simulink model "PulsePairProc_x4"  (Simulink 6.4)
settings: Solver=ode45  StartTime=0.0  StopTime=40000/12e6  RelTol=1e-3
libraries: xbsIndex_r4 x1049, simulink x4, dspsrcs4 x1
(part 1 of 8)
settings Model: LastModifiedBy=tbrimeye

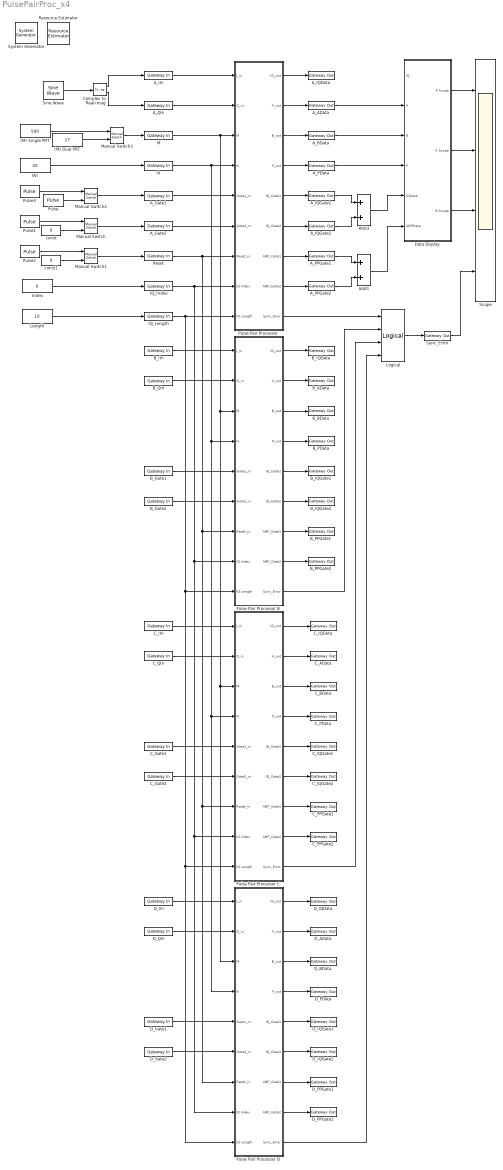
== system PulsePairProc_x4 ==
  " System Generator" : xbsIndex_r4/ System Generator  Tag=genX  SystemSampleTime=-1  xilinxfamily=Virtex4  part=xc4vlx60  speed=-11  package=ff668  synthesis_tool=XST  directory=C:/Work_Projects/Xilinx/SysGen_Outputs/PulsePairProcessor/PulsePairProc_x4_netlist  testbench=off  simulink_period=1/12e6  sysclk_period=(1/12e6)*1e9  incr_netlist=off  trim_vbits=Everywhere in SubSystem  dbl_ovrd=According to Block Masks  core_generation=According to Block Masks  run_coregen=off  deprecated_control=off  eval_field=0  block_type=sysgen
      settings: block_version=8.2
  (M) Dual PRT : Constant  Value=27  OutDataType=sfix(16)  ConRadixGroup=Use specified scaling  OutScaling=2^0  SampleTime=inf  FramePeriod=inf
  (M) Single PRT : Constant  Value=500  OutDataType=sfix(16)  ConRadixGroup=Use specified scaling  OutScaling=2^0  SampleTime=inf  FramePeriod=inf
  (N) : Constant  Value=20  OutDataType=sfix(16)  ConRadixGroup=Use specified scaling  OutScaling=2^0  SampleTime=inf  FramePeriod=inf
  A_AData : xbsIndex_r4/Gateway Out  hdl_port=on  timing_constraint=None  locs_specified=off  LOCs={}  block_type=gatewayout
      settings: infoedit="Gateway out block.  Converts Xilinx fixed point inputs into ouputs of type Simulink integer, double, or fixed point.<P><P>Hardware notes:  In hardware these blocks become top level output ports or are discarded, depending on how they are configured."  xl_area=[0 0 0 0 32 0 0]  block_version=8.2
  A_BData : xbsIndex_r4/Gateway Out  hdl_port=on  timing_constraint=None  locs_specified=off  LOCs={}  block_type=gatewayout
      settings: infoedit="Gateway out block.  Converts Xilinx fixed point inputs into ouputs of type Simulink integer, double, or fixed point.<P><P>Hardware notes:  In hardware these blocks become top level output ports or are discarded, depending on how they are configured."  xl_area=[0 0 0 0 32 0 0]  block_version=8.2
  A_Gate1 : xbsIndex_r4/Gateway In  arith_type=Boolean  n_bits=18  bin_pt=0  quantization="Round  (unbiased: +/- Inf)"  overflow=Flag as error  period=1/12e6  dbl_ovrd=off  timing_constraint=None  locs_specified=off  LOCs={}  block_type=gatewayin
      settings: infoedit="Gateway in block.  Converts inputs of type Simulink integer, double and fixed point to  Xilinx fixed point type.<P><P>Hardware notes:  In hardware these blocks become top level input ports."  xl_area=[0 0 0 0 1 0 0]  block_version=8.2
  A_Gate2 : xbsIndex_r4/Gateway In  arith_type=Boolean  n_bits=18  bin_pt=0  quantization="Round  (unbiased: +/- Inf)"  overflow=Flag as error  period=1/12e6  dbl_ovrd=off  timing_constraint=None  locs_specified=off  LOCs={}  block_type=gatewayin
      settings: infoedit="Gateway in block.  Converts inputs of type Simulink integer, double and fixed point to  Xilinx fixed point type.<P><P>Hardware notes:  In hardware these blocks become top level input ports."  xl_area=[0 0 0 0 1 0 0]  block_version=8.2
  A_IIn : xbsIndex_r4/Gateway In  arith_type="Signed  (2's comp)"  n_bits=16  bin_pt=15  quantization="Round  (unbiased: +/- Inf)"  overflow=Saturate  period=1/12e6  dbl_ovrd=off  timing_constraint=None  locs_specified=off  LOCs={}  block_type=gatewayin
      settings: infoedit="Gateway in block.  Converts inputs of type Simulink integer, double and fixed point to  Xilinx fixed point type.<P><P>Hardware notes:  In hardware these blocks become top level input ports."  xl_area=[0 0 0 0 16 0 0]  block_version=8.2
  A_IQData : xbsIndex_r4/Gateway Out  hdl_port=on  timing_constraint=None  locs_specified=off  LOCs={}  block_type=gatewayout
      settings: infoedit="Gateway out block.  Converts Xilinx fixed point inputs into ouputs of type Simulink integer, double, or fixed point.<P><P>Hardware notes:  In hardware these blocks become top level output ports or are discarded, depending on how they are configured."  xl_area=[0 0 0 0 32 0 0]  block_version=8.2
  A_IQGate1 : xbsIndex_r4/Gateway Out  hdl_port=on  timing_constraint=None  locs_specified=off  LOCs={}  block_type=gatewayout
      settings: infoedit="Gateway out block.  Converts Xilinx fixed point inputs into ouputs of type Simulink integer, double, or fixed point.<P><P>Hardware notes:  In hardware these blocks become top level output ports or are discarded, depending on how they are configured."  xl_area=[0 0 0 0 32 0 0]  block_version=8.2
  A_IQGate2 : xbsIndex_r4/Gateway Out  hdl_port=on  timing_constraint=None  locs_specified=off  LOCs={}  block_type=gatewayout
      settings: infoedit="Gateway out block.  Converts Xilinx fixed point inputs into ouputs of type Simulink integer, double, or fixed point.<P><P>Hardware notes:  In hardware these blocks become top level output ports or are discarded, depending on how they are configured."  xl_area=[0 0 0 0 32 0 0]  block_version=8.2
  A_PData : xbsIndex_r4/Gateway Out  hdl_port=on  timing_constraint=None  locs_specified=off  LOCs={}  block_type=gatewayout
      settings: infoedit="Gateway out block.  Converts Xilinx fixed point inputs into ouputs of type Simulink integer, double, or fixed point.<P><P>Hardware notes:  In hardware these blocks become top level output ports or are discarded, depending on how they are configured."  xl_area=[0 0 0 0 32 0 0]  block_version=8.2
  A_PPGate1 : xbsIndex_r4/Gateway Out  hdl_port=on  timing_constraint=None  locs_specified=off  LOCs={}  block_type=gatewayout
      settings: infoedit="Gateway out block.  Converts Xilinx fixed point inputs into ouputs of type Simulink integer, double, or fixed point.<P><P>Hardware notes:  In hardware these blocks become top level output ports or are discarded, depending on how they are configured."  xl_area=[0 0 0 0 32 0 0]  block_version=8.2
  A_PPGate2 : xbsIndex_r4/Gateway Out  hdl_port=on  timing_constraint=None  locs_specified=off  LOCs={}  block_type=gatewayout
      settings: infoedit="Gateway out block.  Converts Xilinx fixed point inputs into ouputs of type Simulink integer, double, or fixed point.<P><P>Hardware notes:  In hardware these blocks become top level output ports or are discarded, depending on how they are configured."  xl_area=[0 0 0 0 32 0 0]  block_version=8.2
  A_QIn : xbsIndex_r4/Gateway In  arith_type="Signed  (2's comp)"  n_bits=16  bin_pt=15  quantization="Round  (unbiased: +/- Inf)"  overflow=Saturate  period=1/12e6  dbl_ovrd=off  timing_constraint=None  locs_specified=off  LOCs={}  block_type=gatewayin
      settings: infoedit="Gateway in block.  Converts inputs of type Simulink integer, double and fixed point to  Xilinx fixed point type.<P><P>Hardware notes:  In hardware these blocks become top level input ports."  xl_area=[0 0 0 0 16 0 0]  block_version=8.2
  Add1 : Sum  OutScaling=2^-10
  Add3 : Sum  OutScaling=2^-10
  B_AData : xbsIndex_r4/Gateway Out  hdl_port=on  timing_constraint=None  locs_specified=off  LOCs={}  block_type=gatewayout
      settings: infoedit="Gateway out block.  Converts Xilinx fixed point inputs into ouputs of type Simulink integer, double, or fixed point.<P><P>Hardware notes:  In hardware these blocks become top level output ports or are discarded, depending on how they are configured."  xl_area=[0 0 0 0 32 0 0]  block_version=8.2
  B_BData : xbsIndex_r4/Gateway Out  hdl_port=on  timing_constraint=None  locs_specified=off  LOCs={}  block_type=gatewayout
      settings: infoedit="Gateway out block.  Converts Xilinx fixed point inputs into ouputs of type Simulink integer, double, or fixed point.<P><P>Hardware notes:  In hardware these blocks become top level output ports or are discarded, depending on how they are configured."  xl_area=[0 0 0 0 32 0 0]  block_version=8.2
  B_Gate1 : xbsIndex_r4/Gateway In  arith_type=Boolean  n_bits=18  bin_pt=0  quantization="Round  (unbiased: +/- Inf)"  overflow=Flag as error  period=1/12e6  dbl_ovrd=off  timing_constraint=None  locs_specified=off  LOCs={}  block_type=gatewayin
      settings: infoedit="Gateway in block.  Converts inputs of type Simulink integer, double and fixed point to  Xilinx fixed point type.<P><P>Hardware notes:  In hardware these blocks become top level input ports."  xl_area=[0 0 0 0 1 0 0]  block_version=8.2
  B_Gate2 : xbsIndex_r4/Gateway In  arith_type=Boolean  n_bits=18  bin_pt=0  quantization="Round  (unbiased: +/- Inf)"  overflow=Flag as error  period=1/12e6  dbl_ovrd=off  timing_constraint=None  locs_specified=off  LOCs={}  block_type=gatewayin
      settings: infoedit="Gateway in block.  Converts inputs of type Simulink integer, double and fixed point to  Xilinx fixed point type.<P><P>Hardware notes:  In hardware these blocks become top level input ports."  xl_area=[0 0 0 0 1 0 0]  block_version=8.2
  B_IIn : xbsIndex_r4/Gateway In  arith_type="Signed  (2's comp)"  n_bits=16  bin_pt=15  quantization="Round  (unbiased: +/- Inf)"  overflow=Saturate  period=1/12e6  dbl_ovrd=off  timing_constraint=None  locs_specified=off  LOCs={}  block_type=gatewayin
      settings: infoedit="Gateway in block.  Converts inputs of type Simulink integer, double and fixed point to  Xilinx fixed point type.<P><P>Hardware notes:  In hardware these blocks become top level input ports."  xl_area=[0 0 0 0 16 0 0]  block_version=8.2
  B_IQData : xbsIndex_r4/Gateway Out  hdl_port=on  timing_constraint=None  locs_specified=off  LOCs={}  block_type=gatewayout
      settings: infoedit="Gateway out block.  Converts Xilinx fixed point inputs into ouputs of type Simulink integer, double, or fixed point.<P><P>Hardware notes:  In hardware these blocks become top level output ports or are discarded, depending on how they are configured."  xl_area=[0 0 0 0 32 0 0]  block_version=8.2
  B_IQGate1 : xbsIndex_r4/Gateway Out  hdl_port=on  timing_constraint=None  locs_specified=off  LOCs={}  block_type=gatewayout
      settings: infoedit="Gateway out block.  Converts Xilinx fixed point inputs into ouputs of type Simulink integer, double, or fixed point.<P><P>Hardware notes:  In hardware these blocks become top level output ports or are discarded, depending on how they are configured."  xl_area=[0 0 0 0 32 0 0]  block_version=8.2
  B_IQGate2 : xbsIndex_r4/Gateway Out  hdl_port=on  timing_constraint=None  locs_specified=off  LOCs={}  block_type=gatewayout
      settings: infoedit="Gateway out block.  Converts Xilinx fixed point inputs into ouputs of type Simulink integer, double, or fixed point.<P><P>Hardware notes:  In hardware these blocks become top level output ports or are discarded, depending on how they are configured."  xl_area=[0 0 0 0 32 0 0]  block_version=8.2
  B_PData : xbsIndex_r4/Gateway Out  hdl_port=on  timing_constraint=None  locs_specified=off  LOCs={}  block_type=gatewayout
      settings: infoedit="Gateway out block.  Converts Xilinx fixed point inputs into ouputs of type Simulink integer, double, or fixed point.<P><P>Hardware notes:  In hardware these blocks become top level output ports or are discarded, depending on how they are configured."  xl_area=[0 0 0 0 32 0 0]  block_version=8.2
  B_PPGate1 : xbsIndex_r4/Gateway Out  hdl_port=on  timing_constraint=None  locs_specified=off  LOCs={}  block_type=gatewayout
      settings: infoedit="Gateway out block.  Converts Xilinx fixed point inputs into ouputs of type Simulink integer, double, or fixed point.<P><P>Hardware notes:  In hardware these blocks become top level output ports or are discarded, depending on how they are configured."  xl_area=[0 0 0 0 32 0 0]  block_version=8.2
  B_PPGate2 : xbsIndex_r4/Gateway Out  hdl_port=on  timing_constraint=None  locs_specified=off  LOCs={}  block_type=gatewayout
      settings: infoedit="Gateway out block.  Converts Xilinx fixed point inputs into ouputs of type Simulink integer, double, or fixed point.<P><P>Hardware notes:  In hardware these blocks become top level output ports or are discarded, depending on how they are configured."  xl_area=[0 0 0 0 32 0 0]  block_version=8.2
  B_QIn : xbsIndex_r4/Gateway In  arith_type="Signed  (2's comp)"  n_bits=16  bin_pt=15  quantization="Round  (unbiased: +/- Inf)"  overflow=Saturate  period=1/12e6  dbl_ovrd=off  timing_constraint=None  locs_specified=off  LOCs={}  block_type=gatewayin
      settings: infoedit="Gateway in block.  Converts inputs of type Simulink integer, double and fixed point to  Xilinx fixed point type.<P><P>Hardware notes:  In hardware these blocks become top level input ports."  xl_area=[0 0 0 0 16 0 0]  block_version=8.2
  C_AData : xbsIndex_r4/Gateway Out  hdl_port=on  timing_constraint=None  locs_specified=off  LOCs={}  block_type=gatewayout
      settings: infoedit="Gateway out block.  Converts Xilinx fixed point inputs into ouputs of type Simulink integer, double, or fixed point.<P><P>Hardware notes:  In hardware these blocks become top level output ports or are discarded, depending on how they are configured."  xl_area=[0 0 0 0 32 0 0]  block_version=8.2
  C_BData : xbsIndex_r4/Gateway Out  hdl_port=on  timing_constraint=None  locs_specified=off  LOCs={}  block_type=gatewayout
      settings: infoedit="Gateway out block.  Converts Xilinx fixed point inputs into ouputs of type Simulink integer, double, or fixed point.<P><P>Hardware notes:  In hardware these blocks become top level output ports or are discarded, depending on how they are configured."  xl_area=[0 0 0 0 32 0 0]  block_version=8.2
  C_Gate1 : xbsIndex_r4/Gateway In  arith_type=Boolean  n_bits=18  bin_pt=0  quantization="Round  (unbiased: +/- Inf)"  overflow=Flag as error  period=1/12e6  dbl_ovrd=off  timing_constraint=None  locs_specified=off  LOCs={}  block_type=gatewayin
      settings: infoedit="Gateway in block.  Converts inputs of type Simulink integer, double and fixed point to  Xilinx fixed point type.<P><P>Hardware notes:  In hardware these blocks become top level input ports."  xl_area=[0 0 0 0 1 0 0]  block_version=8.2
  C_Gate2 : xbsIndex_r4/Gateway In  arith_type=Boolean  n_bits=18  bin_pt=0  quantization="Round  (unbiased: +/- Inf)"  overflow=Flag as error  period=1/12e6  dbl_ovrd=off  timing_constraint=None  locs_specified=off  LOCs={}  block_type=gatewayin
      settings: infoedit="Gateway in block.  Converts inputs of type Simulink integer, double and fixed point to  Xilinx fixed point type.<P><P>Hardware notes:  In hardware these blocks become top level input ports."  xl_area=[0 0 0 0 1 0 0]  block_version=8.2
  C_IIn : xbsIndex_r4/Gateway In  arith_type="Signed  (2's comp)"  n_bits=16  bin_pt=15  quantization="Round  (unbiased: +/- Inf)"  overflow=Saturate  period=1/12e6  dbl_ovrd=off  timing_constraint=None  locs_specified=off  LOCs={}  block_type=gatewayin
      settings: infoedit="Gateway in block.  Converts inputs of type Simulink integer, double and fixed point to  Xilinx fixed point type.<P><P>Hardware notes:  In hardware these blocks become top level input ports."  xl_area=[0 0 0 0 16 0 0]  block_version=8.2
  C_IQData : xbsIndex_r4/Gateway Out  hdl_port=on  timing_constraint=None  locs_specified=off  LOCs={}  block_type=gatewayout
      settings: infoedit="Gateway out block.  Converts Xilinx fixed point inputs into ouputs of type Simulink integer, double, or fixed point.<P><P>Hardware notes:  In hardware these blocks become top level output ports or are discarded, depending on how they are configured."  xl_area=[0 0 0 0 32 0 0]  block_version=8.2
  C_IQGate1 : xbsIndex_r4/Gateway Out  hdl_port=on  timing_constraint=None  locs_specified=off  LOCs={}  block_type=gatewayout
      settings: infoedit="Gateway out block.  Converts Xilinx fixed point inputs into ouputs of type Simulink integer, double, or fixed point.<P><P>Hardware notes:  In hardware these blocks become top level output ports or are discarded, depending on how they are configured."  xl_area=[0 0 0 0 32 0 0]  block_version=8.2
  C_IQGate2 : xbsIndex_r4/Gateway Out  hdl_port=on  timing_constraint=None  locs_specified=off  LOCs={}  block_type=gatewayout
      settings: infoedit="Gateway out block.  Converts Xilinx fixed point inputs into ouputs of type Simulink integer, double, or fixed point.<P><P>Hardware notes:  In hardware these blocks become top level output ports or are discarded, depending on how they are configured."  xl_area=[0 0 0 0 32 0 0]  block_version=8.2
  C_PData : xbsIndex_r4/Gateway Out  hdl_port=on  timing_constraint=None  locs_specified=off  LOCs={}  block_type=gatewayout
      settings: infoedit="Gateway out block.  Converts Xilinx fixed point inputs into ouputs of type Simulink integer, double, or fixed point.<P><P>Hardware notes:  In hardware these blocks become top level output ports or are discarded, depending on how they are configured."  xl_area=[0 0 0 0 32 0 0]  block_version=8.2
  C_PPGate1 : xbsIndex_r4/Gateway Out  hdl_port=on  timing_constraint=None  locs_specified=off  LOCs={}  block_type=gatewayout
      settings: infoedit="Gateway out block.  Converts Xilinx fixed point inputs into ouputs of type Simulink integer, double, or fixed point.<P><P>Hardware notes:  In hardware these blocks become top level output ports or are discarded, depending on how they are configured."  xl_area=[0 0 0 0 32 0 0]  block_version=8.2
  C_PPGate2 : xbsIndex_r4/Gateway Out  hdl_port=on  timing_constraint=None  locs_specified=off  LOCs={}  block_type=gatewayout
      settings: infoedit="Gateway out block.  Converts Xilinx fixed point inputs into ouputs of type Simulink integer, double, or fixed point.<P><P>Hardware notes:  In hardware these blocks become top level output ports or are discarded, depending on how they are configured."  xl_area=[0 0 0 0 32 0 0]  block_version=8.2
  C_QIn : xbsIndex_r4/Gateway In  arith_type="Signed  (2's comp)"  n_bits=16  bin_pt=15  quantization="Round  (unbiased: +/- Inf)"  overflow=Saturate  period=1/12e6  dbl_ovrd=off  timing_constraint=None  locs_specified=off  LOCs={}  block_type=gatewayin
      settings: infoedit="Gateway in block.  Converts inputs of type Simulink integer, double and fixed point to  Xilinx fixed point type.<P><P>Hardware notes:  In hardware these blocks become top level input ports."  xl_area=[0 0 0 0 16 0 0]  block_version=8.2
  Complex to Real-Imag : ComplexToRealImag
  D_AData : xbsIndex_r4/Gateway Out  hdl_port=on  timing_constraint=None  locs_specified=off  LOCs={}  block_type=gatewayout
      settings: infoedit="Gateway out block.  Converts Xilinx fixed point inputs into ouputs of type Simulink integer, double, or fixed point.<P><P>Hardware notes:  In hardware these blocks become top level output ports or are discarded, depending on how they are configured."  xl_area=[0 0 0 0 32 0 0]  block_version=8.2
  D_BData : xbsIndex_r4/Gateway Out  hdl_port=on  timing_constraint=None  locs_specified=off  LOCs={}  block_type=gatewayout
      settings: infoedit="Gateway out block.  Converts Xilinx fixed point inputs into ouputs of type Simulink integer, double, or fixed point.<P><P>Hardware notes:  In hardware these blocks become top level output ports or are discarded, depending on how they are configured."  xl_area=[0 0 0 0 32 0 0]  block_version=8.2
  D_Gate1 : xbsIndex_r4/Gateway In  arith_type=Boolean  n_bits=18  bin_pt=0  quantization="Round  (unbiased: +/- Inf)"  overflow=Flag as error  period=1/12e6  dbl_ovrd=off  timing_constraint=None  locs_specified=off  LOCs={}  block_type=gatewayin
      settings: infoedit="Gateway in block.  Converts inputs of type Simulink integer, double and fixed point to  Xilinx fixed point type.<P><P>Hardware notes:  In hardware these blocks become top level input ports."  xl_area=[0 0 0 0 1 0 0]  block_version=8.2
  D_Gate2 : xbsIndex_r4/Gateway In  arith_type=Boolean  n_bits=18  bin_pt=0  quantization="Round  (unbiased: +/- Inf)"  overflow=Flag as error  period=1/12e6  dbl_ovrd=off  timing_constraint=None  locs_specified=off  LOCs={}  block_type=gatewayin
      settings: infoedit="Gateway in block.  Converts inputs of type Simulink integer, double and fixed point to  Xilinx fixed point type.<P><P>Hardware notes:  In hardware these blocks become top level input ports."  xl_area=[0 0 0 0 1 0 0]  block_version=8.2
  D_IIn : xbsIndex_r4/Gateway In  arith_type="Signed  (2's comp)"  n_bits=16  bin_pt=15  quantization="Round  (unbiased: +/- Inf)"  overflow=Saturate  period=1/12e6  dbl_ovrd=off  timing_constraint=None  locs_specified=off  LOCs={}  block_type=gatewayin
      settings: infoedit="Gateway in block.  Converts inputs of type Simulink integer, double and fixed point to  Xilinx fixed point type.<P><P>Hardware notes:  In hardware these blocks become top level input ports."  xl_area=[0 0 0 0 16 0 0]  block_version=8.2
  D_IQData : xbsIndex_r4/Gateway Out  hdl_port=on  timing_constraint=None  locs_specified=off  LOCs={}  block_type=gatewayout
      settings: infoedit="Gateway out block.  Converts Xilinx fixed point inputs into ouputs of type Simulink integer, double, or fixed point.<P><P>Hardware notes:  In hardware these blocks become top level output ports or are discarded, depending on how they are configured."  xl_area=[0 0 0 0 32 0 0]  block_version=8.2
  D_IQGate1 : xbsIndex_r4/Gateway Out  hdl_port=on  timing_constraint=None  locs_specified=off  LOCs={}  block_type=gatewayout
      settings: infoedit="Gateway out block.  Converts Xilinx fixed point inputs into ouputs of type Simulink integer, double, or fixed point.<P><P>Hardware notes:  In hardware these blocks become top level output ports or are discarded, depending on how they are configured."  xl_area=[0 0 0 0 32 0 0]  block_version=8.2
  D_IQGate2 : xbsIndex_r4/Gateway Out  hdl_port=on  timing_constraint=None  locs_specified=off  LOCs={}  block_type=gatewayout
      settings: infoedit="Gateway out block.  Converts Xilinx fixed point inputs into ouputs of type Simulink integer, double, or fixed point.<P><P>Hardware notes:  In hardware these blocks become top level output ports or are discarded, depending on how they are configured."  xl_area=[0 0 0 0 32 0 0]  block_version=8.2
  D_PData : xbsIndex_r4/Gateway Out  hdl_port=on  timing_constraint=None  locs_specified=off  LOCs={}  block_type=gatewayout
      settings: infoedit="Gateway out block.  Converts Xilinx fixed point inputs into ouputs of type Simulink integer, double, or fixed point.<P><P>Hardware notes:  In hardware these blocks become top level output ports or are discarded, depending on how they are configured."  xl_area=[0 0 0 0 32 0 0]  block_version=8.2
  D_PPGate1 : xbsIndex_r4/Gateway Out  hdl_port=on  timing_constraint=None  locs_specified=off  LOCs={}  block_type=gatewayout
      settings: infoedit="Gateway out block.  Converts Xilinx fixed point inputs into ouputs of type Simulink integer, double, or fixed point.<P><P>Hardware notes:  In hardware these blocks become top level output ports or are discarded, depending on how they are configured."  xl_area=[0 0 0 0 32 0 0]  block_version=8.2
  D_PPGate2 : xbsIndex_r4/Gateway Out  hdl_port=on  timing_constraint=None  locs_specified=off  LOCs={}  block_type=gatewayout
      settings: infoedit="Gateway out block.  Converts Xilinx fixed point inputs into ouputs of type Simulink integer, double, or fixed point.<P><P>Hardware notes:  In hardware these blocks become top level output ports or are discarded, depending on how they are configured."  xl_area=[0 0 0 0 32 0 0]  block_version=8.2
  D_QIn : xbsIndex_r4/Gateway In  arith_type="Signed  (2's comp)"  n_bits=16  bin_pt=15  quantization="Round  (unbiased: +/- Inf)"  overflow=Saturate  period=1/12e6  dbl_ovrd=off  timing_constraint=None  locs_specified=off  LOCs={}  block_type=gatewayin
      settings: infoedit="Gateway in block.  Converts inputs of type Simulink integer, double and fixed point to  Xilinx fixed point type.<P><P>Hardware notes:  In hardware these blocks become top level input ports."  xl_area=[0 0 0 0 16 0 0]  block_version=8.2
  Data Display : Subsystem
  IQ_Index : xbsIndex_r4/Gateway In  arith_type=Unsigned  n_bits=10  bin_pt=0  quantization="Round  (unbiased: +/- Inf)"  overflow=Flag as error  period=1/12e6  dbl_ovrd=off  timing_constraint=None  locs_specified=off  LOCs={}  block_type=gatewayin
      settings: infoedit="Gateway in block.  Converts inputs of type Simulink integer, double and fixed point to  Xilinx fixed point type.<P><P>Hardware notes:  In hardware these blocks become top level input ports."  xl_area=[0 0 0 0 11 0 0]  block_version=8.2
  IQ_Length : xbsIndex_r4/Gateway In  arith_type=Unsigned  n_bits=10  bin_pt=0  quantization="Round  (unbiased: +/- Inf)"  overflow=Flag as error  period=1/12e6  dbl_ovrd=off  timing_constraint=None  locs_specified=off  LOCs={}  block_type=gatewayin
      settings: infoedit="Gateway in block.  Converts inputs of type Simulink integer, double and fixed point to  Xilinx fixed point type.<P><P>Hardware notes:  In hardware these blocks become top level input ports."  xl_area=[0 0 0 0 11 0 0]  block_version=8.2
  Index : Constant  Value=0  OutDataType=sfix(16)  ConRadixGroup=Use specified scaling  OutScaling=2^0  SampleTime=inf  FramePeriod=inf
  Length : Constant  Value=10  OutDataType=sfix(16)  ConRadixGroup=Use specified scaling  OutScaling=2^0  SampleTime=inf  FramePeriod=inf
  Logical : xbsIndex_r4/Logical  logical_function=OR  inputs=4  en=off  latency=0  precision=Full  arith_type=Unsigned  n_bits=16  bin_pt=0  align_bp=on  dbl_ovrd=off  block_type=logical
      settings: block_version=8.2
  M : xbsIndex_r4/Gateway In  arith_type=Unsigned  n_bits=10  bin_pt=0  quantization="Round  (unbiased: +/- Inf)"  overflow=Flag as error  period=1/12e6  dbl_ovrd=off  timing_constraint=None  locs_specified=off  LOCs={}  block_type=gatewayin
      settings: infoedit="Gateway in block.  Converts inputs of type Simulink integer, double and fixed point to  Xilinx fixed point type.<P><P>Hardware notes:  In hardware these blocks become top level input ports."  xl_area=[0 0 0 0 11 0 0]  block_version=8.2
  Manual Switch : simulink/Signal Routing/Manual Switch  SystemSampleTime=-1  sw=0  action=0
  Manual Switch1 : simulink/Signal Routing/Manual Switch  SystemSampleTime=-1  sw=0  action=0
  Manual Switch2 : simulink/Signal Routing/Manual Switch  SystemSampleTime=-1  sw=1  action=0
  Manual Switch3 : simulink/Signal Routing/Manual Switch  SystemSampleTime=-1  sw=1  action=0
  N : xbsIndex_r4/Gateway In  arith_type=Unsigned  n_bits=7  bin_pt=0  quantization="Round  (unbiased: +/- Inf)"  overflow=Flag as error  period=1/12e6  dbl_ovrd=off  timing_constraint=None  locs_specified=off  LOCs={}  block_type=gatewayin
      settings: infoedit="Gateway in block.  Converts inputs of type Simulink integer, double and fixed point to  Xilinx fixed point type.<P><P>Hardware notes:  In hardware these blocks become top level input ports."  xl_area=[0 0 0 0 7 0 0]  block_version=8.2
  Pulse : DiscretePulseGenerator  PulseType=Time based  Period=900/40e6  PulseWidth=10  PhaseDelay=0*100/12e6
  Pulse Pair Processor : Subsystem
  Pulse Pair Processor B : Subsystem
  Pulse Pair Processor C : Subsystem
  Pulse Pair Processor D : Subsystem
  Pulse1 : DiscretePulseGenerator  PulseType=Time based  Period=900/40e6  PulseWidth=10  PhaseDelay=150/12e6
  Pulse2 : DiscretePulseGenerator  PulseType=Time based  Period=5000/12e6  PhaseDelay=600/12e6
  Pulse3 : DiscretePulseGenerator  PulseType=Time based  Period=625/12e6  PulseWidth=80  PhaseDelay=0/12e6
  Reset : xbsIndex_r4/Gateway In  arith_type=Boolean  n_bits=18  bin_pt=0  quantization="Round  (unbiased: +/- Inf)"  overflow=Flag as error  period=1/12e6  dbl_ovrd=off  timing_constraint=None  locs_specified=off  LOCs={}  block_type=gatewayin
      settings: infoedit="Gateway in block.  Converts inputs of type Simulink integer, double and fixed point to  Xilinx fixed point type.<P><P>Hardware notes:  In hardware these blocks become top level input ports."  xl_area=[0 0 0 0 1 0 0]  block_version=8.2
  Resource Estimator : xbsIndex_r4/Resource Estimator  Tag=resEstTag  Slices=813  FFs=745  BRAMs=24  LUTs=1307  IOBs=244  EBMs=6  TBUFs=0  xl_use_estimator_area=off  est_options=Post Map  xl_estimator_area=[1915 2342 0 3405 33 4 0]  block_type=resource_estimator
      settings: AttributesFormatString=Resource\nEstimator  block_version=8.2
  Scope : Scope  NumInputPorts=4
      settings: TimeRange=0.0002083333333333334  YMin=-1~-5~-5~-5  YMax=1~5~5~5  MaxDataPoints=5000000
  Sine Wave : dspsrcs4/Sine Wave  Amplitude=.99  Frequency=10e3  Phase=0  SampleMode=Discrete  OutComplex=Complex  CompMethod=Trigonometric fcn  TableSize=Speed  SampleTime=1/12e6  SamplesPerFrame=1  dataType=double  wordLen=16  udDataType=sfix(16)  fracBitsMode=Best precision  numFracBits=15  ResetState=Restart at time zero
  Sync_Error : xbsIndex_r4/Gateway Out  hdl_port=on  timing_constraint=None  locs_specified=off  LOCs={}  block_type=gatewayout
      settings: infoedit="Gateway out block.  Converts Xilinx fixed point inputs into ouputs of type Simulink integer, double, or fixed point.<P><P>Hardware notes:  In hardware these blocks become top level output ports or are discarded, depending on how they are configured."  xl_area=[0 0 0 0 32 0 0]  block_version=8.2
  const : Constant  Value=0  OutDataType=sfix(16)  ConRadixGroup=Use specified scaling  OutScaling=2^0  SampleTime=inf  FramePeriod=inf
  const1 : Constant  Value=0  OutDataType=sfix(16)  ConRadixGroup=Use specified scaling  OutScaling=2^0  SampleTime=inf  FramePeriod=inf
  wires:
  A_IIn/1 -> Pulse Pair Processor/1(I_in)
  A_QIn/1 -> Pulse Pair Processor/2(Q_in)
  (N)/1 -> N/1
  M/1 -> Pulse Pair Processor D/3(M), Pulse Pair Processor C/3(M), Pulse Pair Processor B/3(M), Pulse Pair Processor/3(M)
  N/1 -> Pulse Pair Processor D/4(N), Pulse Pair Processor C/4(N), Pulse Pair Processor B/4(N), Pulse Pair Processor/4(N)
  Pulse1/1 -> Manual Switch/1
  const/1 -> Manual Switch/2
  Manual Switch/1 -> A_Gate2/1
  A_Gate1/1 -> Pulse Pair Processor/5(Gate1_in)
  A_Gate2/1 -> Pulse Pair Processor/6(Gate2_in)
  Pulse Pair Processor/2(A_out) -> A_AData/1
  Pulse Pair Processor/3(B_out) -> A_BData/1
  Pulse Pair Processor/4(P_out) -> A_PData/1
  Data Display/1(P Scope) -> Scope/1
  Data Display/2(A Scope) -> Scope/2
  Data Display/3(B Scope) -> Scope/3
  Pulse Pair Processor/1(IQ_out) -> A_IQData/1
  Pulse Pair Processor/5(IQ_Gate1) -> A_IQGate1/1
  Pulse Pair Processor/6(IQ_Gate2) -> A_IQGate2/1
  A_IQGate1/1 -> Add3/1
  A_IQGate2/1 -> Add3/2
  Pulse Pair Processor/7(ABP_Gate1) -> A_PPGate1/1
  Pulse Pair Processor/8(ABP_Gate2) -> A_PPGate2/1
  A_PData/1 -> Data Display/4(P)
  Reset/1 -> Pulse Pair Processor D/7(Reset_in), Pulse Pair Processor C/7(Reset_in), Pulse Pair Processor B/7(Reset_in), Pulse Pair Processor/7(Reset_in)
  Pulse2/1 -> Manual Switch1/1
  const1/1 -> Manual Switch1/2
  Manual Switch1/1 -> Reset/1
  A_AData/1 -> Data Display/2(A)
  A_BData/1 -> Data Display/3(B)
  A_PPGate1/1 -> Add1/1
  A_PPGate2/1 -> Add1/2
  Add1/1 -> Data Display/6(ABPGate)
  Sine Wave/1 -> Complex to Real-Imag/1
  Complex to Real-Imag/1 -> A_IIn/1
  Complex to Real-Imag/2 -> A_QIn/1
  Add3/1 -> Data Display/5(IQGate)
  IQ_Index/1 -> Pulse Pair Processor D/8(IQ Index), Pulse Pair Processor C/8(IQ Index), Pulse Pair Processor B/8(IQ Index), Pulse Pair Processor/8(IQ Index)
  IQ_Length/1 -> Pulse Pair Processor D/9(IQ Length), Pulse Pair Processor C/9(IQ Length), Pulse Pair Processor B/9(IQ Length), Pulse Pair Processor/9(IQ Length)
  Index/1 -> IQ_Index/1
  Length/1 -> IQ_Length/1
  B_IIn/1 -> Pulse Pair Processor B/1(I_in)
  B_QIn/1 -> Pulse Pair Processor B/2(Q_in)
  C_IIn/1 -> Pulse Pair Processor C/1(I_in)
  C_QIn/1 -> Pulse Pair Processor C/2(Q_in)
  D_IIn/1 -> Pulse Pair Processor D/1(I_in)
  D_QIn/1 -> Pulse Pair Processor D/2(Q_in)
  B_Gate1/1 -> Pulse Pair Processor B/5(Gate1_in)
  B_Gate2/1 -> Pulse Pair Processor B/6(Gate2_in)
  C_Gate1/1 -> Pulse Pair Processor C/5(Gate1_in)
  C_Gate2/1 -> Pulse Pair Processor C/6(Gate2_in)
  D_Gate1/1 -> Pulse Pair Processor D/5(Gate1_in)
  D_Gate2/1 -> Pulse Pair Processor D/6(Gate2_in)
  Pulse Pair Processor B/2(A_out) -> B_AData/1
  Pulse Pair Processor B/3(B_out) -> B_BData/1
  Pulse Pair Processor B/4(P_out) -> B_PData/1
  Pulse Pair Processor B/1(IQ_out) -> B_IQData/1
  Pulse Pair Processor B/5(IQ_Gate1) -> B_IQGate1/1
  Pulse Pair Processor B/6(IQ_Gate2) -> B_IQGate2/1
  Pulse Pair Processor B/7(ABP_Gate1) -> B_PPGate1/1
  Pulse Pair Processor B/8(ABP_Gate2) -> B_PPGate2/1
  Pulse Pair Processor C/2(A_out) -> C_AData/1
  Pulse Pair Processor C/3(B_out) -> C_BData/1
  Pulse Pair Processor C/4(P_out) -> C_PData/1
  Pulse Pair Processor C/1(IQ_out) -> C_IQData/1
  Pulse Pair Processor C/5(IQ_Gate1) -> C_IQGate1/1
  Pulse Pair Processor C/6(IQ_Gate2) -> C_IQGate2/1
  Pulse Pair Processor C/7(ABP_Gate1) -> C_PPGate1/1
  Pulse Pair Processor C/8(ABP_Gate2) -> C_PPGate2/1
  Pulse Pair Processor D/2(A_out) -> D_AData/1
  Pulse Pair Processor D/3(B_out) -> D_BData/1
  Pulse Pair Processor D/4(P_out) -> D_PData/1
  Pulse Pair Processor D/1(IQ_out) -> D_IQData/1
  Pulse Pair Processor D/5(IQ_Gate1) -> D_IQGate1/1
  Pulse Pair Processor D/6(IQ_Gate2) -> D_IQGate2/1
  Pulse Pair Processor D/7(ABP_Gate1) -> D_PPGate1/1
  Pulse Pair Processor D/8(ABP_Gate2) -> D_PPGate2/1
  Pulse Pair Processor/9(Sync_Error) -> Logical/1
  Pulse Pair Processor B/9(Sync_Error) -> Logical/2
  Pulse Pair Processor C/9(Sync_Error) -> Logical/3
  Pulse Pair Processor D/9(Sync_Error) -> Logical/4
  Logical/1 -> Sync_Error/1
  Sync_Error/1 -> Scope/4
  Manual Switch2/1 -> A_Gate1/1
  Pulse3/1 -> Manual Switch2/1
  Pulse/1 -> Manual Switch2/2
  Manual Switch3/1 -> M/1
  (M) Single PRT/1 -> Manual Switch3/1
  (M) Dual PRT/1 -> Manual Switch3/2

== system PulsePairProc_x4/Data Display ==
  IQ : Inport
  A : Inport  Port=2
  B : Inport  Port=3
  P : Inport  Port=4
  IQGate : Inport  Port=5
  ABPGate : Inport  Port=6
  Mux : Mux
  Mux1 : Mux
  Mux2 : Mux
  P Scope : Outport
  A Scope : Outport  Port=2
  B Scope : Outport  Port=3
  wires:
  IQ/1 -> Mux/1, Mux1/1, Mux2/1
  Mux/1 -> P Scope/1
  Mux1/1 -> A Scope/1
  Mux2/1 -> B Scope/1
  P/1 -> Mux/2
  IQGate/1 -> Mux1/2, Mux2/2, Mux/3
  ABPGate/1 -> Mux1/4, Mux2/4, Mux/4
  A/1 -> Mux1/3
  B/1 -> Mux2/3

== system PulsePairProc_x4/Pulse Pair Processor ==
  I_in : Inport
  Q_in : Inport  Port=2
  M : Inport  Port=3
  N : Inport  Port=4
  Gate1_in : Inport  Port=5
  Gate2_in : Inport  Port=6
  Reset_in : Inport  Port=7
  IQ Index : Inport  Port=8
  IQ Length : Inport  Port=9
  Calc : Subsystem
  Sum : Subsystem
  IQ_out : Outport
  A_out : Outport  Port=2
  B_out : Outport  Port=3
  P_out : Outport  Port=4
  IQ_Gate1 : Outport  Port=5
  IQ_Gate2 : Outport  Port=6
  ABP_Gate1 : Outport  Port=7
  ABP_Gate2 : Outport  Port=8
  Sync_Error : Outport  Port=9
  wires:
  Calc/2(A Data) -> Sum/2(A_Data_In)
  Calc/3(B_Data) -> Sum/3(B_Data_In)
  Calc/4(P_Data) -> Sum/4(P_Data_In)
  Calc/5(M_Out) -> Sum/5(M)
  Calc/6(N_Out) -> Sum/6(N)
  Calc/7(Gate1_Out) -> Sum/7(Gate 1)
  Calc/8(Gate2_Out) -> Sum/8(Gate 2)
  Calc/1(IQ_Data) -> Sum/1(IQ_Data_In)
  Calc/9(Reset_Out) -> Sum/9(Reset)
  Sum/1(IQ) -> IQ_out/1
  I_in/1 -> Calc/1(I)
  Q_in/1 -> Calc/2(Q)
  M/1 -> Calc/3(M)
  N/1 -> Calc/4(N)
  Gate1_in/1 -> Calc/5(Gate1_In)
  Sum/5(IQ Gate 1) -> IQ_Gate1/1
  Sum/6(IQ Gate 2) -> IQ_Gate2/1
  Gate2_in/1 -> Calc/6(Gate2_In)
  Sum/7(PP Gate 1) -> ABP_Gate1/1
  Reset_in/1 -> Calc/7(Reset_In)
  Sum/8(PP Gate 2) -> ABP_Gate2/1
  Sum/2(A Data) -> A_out/1
  Sum/3(B Data) -> B_out/1
  Sum/4(P Data) -> P_out/1
  IQ Index/1 -> Calc/8(IQ Index)
  IQ Length/1 -> Calc/9(IQ Length)
  Calc/10(IQ Index_Out) -> Sum/10(IQ Index)
  Calc/11(IQ Length_Out) -> Sum/11(IQ Length)
  Sum/9(Sync Error) -> Sync_Error/1

== system PulsePairProc_x4/Pulse Pair Processor B ==
  I_in : Inport
  Q_in : Inport  Port=2
  M : Inport  Port=3
  N : Inport  Port=4
  Gate1_in : Inport  Port=5
  Gate2_in : Inport  Port=6
  Reset_in : Inport  Port=7
  IQ Index : Inport  Port=8
  IQ Length : Inport  Port=9
  Calc : Subsystem
  Sum : Subsystem
  IQ_out : Outport
  A_out : Outport  Port=2
  B_out : Outport  Port=3
  P_out : Outport  Port=4
  IQ_Gate1 : Outport  Port=5
  IQ_Gate2 : Outport  Port=6
  ABP_Gate1 : Outport  Port=7
  ABP_Gate2 : Outport  Port=8
  Sync_Error : Outport  Port=9
  wires:
  Calc/2(A Data) -> Sum/2(A_Data_In)
  Calc/3(B_Data) -> Sum/3(B_Data_In)
  Calc/4(P_Data) -> Sum/4(P_Data_In)
  Calc/5(M_Out) -> Sum/5(M)
  Calc/6(N_Out) -> Sum/6(N)
  Calc/7(Gate1_Out) -> Sum/7(Gate 1)
  Calc/8(Gate2_Out) -> Sum/8(Gate 2)
  Calc/1(IQ_Data) -> Sum/1(IQ_Data_In)
  Calc/9(Reset_Out) -> Sum/9(Reset)
  Sum/1(IQ) -> IQ_out/1
  I_in/1 -> Calc/1(I)
  Q_in/1 -> Calc/2(Q)
  M/1 -> Calc/3(M)
  N/1 -> Calc/4(N)
  Gate1_in/1 -> Calc/5(Gate1_In)
  Sum/5(IQ Gate 1) -> IQ_Gate1/1
  Sum/6(IQ Gate 2) -> IQ_Gate2/1
  Gate2_in/1 -> Calc/6(Gate2_In)
  Sum/7(PP Gate 1) -> ABP_Gate1/1
  Reset_in/1 -> Calc/7(Reset_In)
  Sum/8(PP Gate 2) -> ABP_Gate2/1
  Sum/2(A Data) -> A_out/1
  Sum/3(B Data) -> B_out/1
  Sum/4(P Data) -> P_out/1
  IQ Index/1 -> Calc/8(IQ Index)
  IQ Length/1 -> Calc/9(IQ Length)
  Calc/10(IQ Index_Out) -> Sum/10(IQ Index)
  Calc/11(IQ Length_Out) -> Sum/11(IQ Length)
  Sum/9(Sync Error) -> Sync_Error/1

== system PulsePairProc_x4/Pulse Pair Processor C ==
  I_in : Inport
  Q_in : Inport  Port=2
  M : Inport  Port=3
  N : Inport  Port=4
  Gate1_in : Inport  Port=5
  Gate2_in : Inport  Port=6
  Reset_in : Inport  Port=7
  IQ Index : Inport  Port=8
  IQ Length : Inport  Port=9
  Calc : Subsystem
  Sum : Subsystem
  IQ_out : Outport
  A_out : Outport  Port=2
  B_out : Outport  Port=3
  P_out : Outport  Port=4
  IQ_Gate1 : Outport  Port=5
  IQ_Gate2 : Outport  Port=6
  ABP_Gate1 : Outport  Port=7
  ABP_Gate2 : Outport  Port=8
  Sync_Error : Outport  Port=9
  wires:
  Calc/2(A Data) -> Sum/2(A_Data_In)
  Calc/3(B_Data) -> Sum/3(B_Data_In)
  Calc/4(P_Data) -> Sum/4(P_Data_In)
  Calc/5(M_Out) -> Sum/5(M)
  Calc/6(N_Out) -> Sum/6(N)
  Calc/7(Gate1_Out) -> Sum/7(Gate 1)
  Calc/8(Gate2_Out) -> Sum/8(Gate 2)
  Calc/1(IQ_Data) -> Sum/1(IQ_Data_In)
  Calc/9(Reset_Out) -> Sum/9(Reset)
  Sum/1(IQ) -> IQ_out/1
  I_in/1 -> Calc/1(I)
  Q_in/1 -> Calc/2(Q)
  M/1 -> Calc/3(M)
  N/1 -> Calc/4(N)
  Gate1_in/1 -> Calc/5(Gate1_In)
  Sum/5(IQ Gate 1) -> IQ_Gate1/1
  Sum/6(IQ Gate 2) -> IQ_Gate2/1
  Gate2_in/1 -> Calc/6(Gate2_In)
  Sum/7(PP Gate 1) -> ABP_Gate1/1
  Reset_in/1 -> Calc/7(Reset_In)
  Sum/8(PP Gate 2) -> ABP_Gate2/1
  Sum/2(A Data) -> A_out/1
  Sum/3(B Data) -> B_out/1
  Sum/4(P Data) -> P_out/1
  IQ Index/1 -> Calc/8(IQ Index)
  IQ Length/1 -> Calc/9(IQ Length)
  Calc/10(IQ Index_Out) -> Sum/10(IQ Index)
  Calc/11(IQ Length_Out) -> Sum/11(IQ Length)
  Sum/9(Sync Error) -> Sync_Error/1

== system PulsePairProc_x4/Pulse Pair Processor D ==
  I_in : Inport
  Q_in : Inport  Port=2
  M : Inport  Port=3
  N : Inport  Port=4
  Gate1_in : Inport  Port=5
  Gate2_in : Inport  Port=6
  Reset_in : Inport  Port=7
  IQ Index : Inport  Port=8
  IQ Length : Inport  Port=9
  Calc : Subsystem
  Sum : Subsystem
  IQ_out : Outport
  A_out : Outport  Port=2
  B_out : Outport  Port=3
  P_out : Outport  Port=4
  IQ_Gate1 : Outport  Port=5
  IQ_Gate2 : Outport  Port=6
  ABP_Gate1 : Outport  Port=7
  ABP_Gate2 : Outport  Port=8
  Sync_Error : Outport  Port=9
  wires:
  Calc/2(A Data) -> Sum/2(A_Data_In)
  Calc/3(B_Data) -> Sum/3(B_Data_In)
  Calc/4(P_Data) -> Sum/4(P_Data_In)
  Calc/5(M_Out) -> Sum/5(M)
  Calc/6(N_Out) -> Sum/6(N)
  Calc/7(Gate1_Out) -> Sum/7(Gate 1)
  Calc/8(Gate2_Out) -> Sum/8(Gate 2)
  Calc/1(IQ_Data) -> Sum/1(IQ_Data_In)
  Calc/9(Reset_Out) -> Sum/9(Reset)
  Sum/1(IQ) -> IQ_out/1
  I_in/1 -> Calc/1(I)
  Q_in/1 -> Calc/2(Q)
  M/1 -> Calc/3(M)
  N/1 -> Calc/4(N)
  Gate1_in/1 -> Calc/5(Gate1_In)
  Sum/5(IQ Gate 1) -> IQ_Gate1/1
  Sum/6(IQ Gate 2) -> IQ_Gate2/1
  Gate2_in/1 -> Calc/6(Gate2_In)
  Sum/7(PP Gate 1) -> ABP_Gate1/1
  Reset_in/1 -> Calc/7(Reset_In)
  Sum/8(PP Gate 2) -> ABP_Gate2/1
  Sum/2(A Data) -> A_out/1
  Sum/3(B Data) -> B_out/1
  Sum/4(P Data) -> P_out/1
  IQ Index/1 -> Calc/8(IQ Index)
  IQ Length/1 -> Calc/9(IQ Length)
  Calc/10(IQ Index_Out) -> Sum/10(IQ Index)
  Calc/11(IQ Length_Out) -> Sum/11(IQ Length)
  Sum/9(Sync Error) -> Sync_Error/1

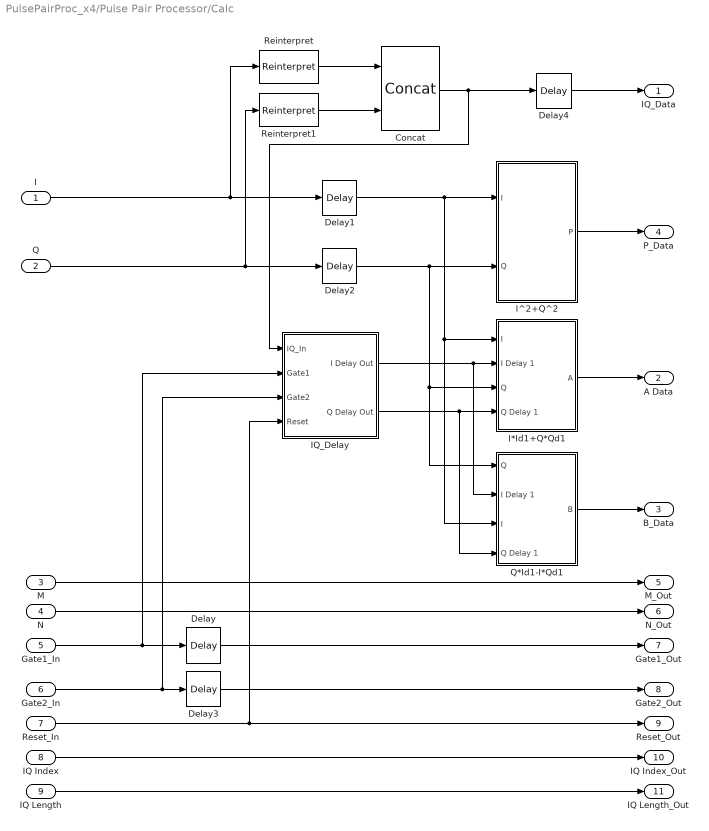
== system PulsePairProc_x4/Pulse Pair Processor/Calc ==
  I : Inport
  Q : Inport  Port=2
  M : Inport  Port=3
  N : Inport  Port=4
  Gate1_In : Inport  Port=5
  Gate2_In : Inport  Port=6
  Reset_In : Inport  Port=7
  IQ Index : Inport  Port=8
  IQ Length : Inport  Port=9
  Concat : xbsIndex_r4/Concat  num_inputs=2  dbl_ovrd=off  block_type=concat
      settings: block_version=8.2
  Delay : xbsIndex_r4/Delay  en=off  latency=6  dbl_ovrd=off  reg_retiming=off  block_type=delay
      settings: infoedit=Hardware notes: A delay line is a chain, each link of which is an SRL16 followed by a flip-flop. If register retiming is enabled, the delay line is a chain of flip-flops.  block_version=8.2
  Delay1 : xbsIndex_r4/Delay  en=off  latency=4  dbl_ovrd=off  reg_retiming=off  block_type=delay
      settings: infoedit=Hardware notes: A delay line is a chain, each link of which is an SRL16 followed by a flip-flop. If register retiming is enabled, the delay line is a chain of flip-flops.  block_version=8.2
  Delay2 : xbsIndex_r4/Delay  en=off  latency=4  dbl_ovrd=off  reg_retiming=off  block_type=delay
      settings: infoedit=Hardware notes: A delay line is a chain, each link of which is an SRL16 followed by a flip-flop. If register retiming is enabled, the delay line is a chain of flip-flops.  block_version=8.2
  Delay3 : xbsIndex_r4/Delay  en=off  latency=6  dbl_ovrd=off  reg_retiming=off  block_type=delay
      settings: infoedit=Hardware notes: A delay line is a chain, each link of which is an SRL16 followed by a flip-flop. If register retiming is enabled, the delay line is a chain of flip-flops.  block_version=8.2
  Delay4 : xbsIndex_r4/Delay  en=off  latency=6  dbl_ovrd=off  reg_retiming=off  block_type=delay
      settings: infoedit=Hardware notes: A delay line is a chain, each link of which is an SRL16 followed by a flip-flop. If register retiming is enabled, the delay line is a chain of flip-flops.  block_version=8.2
  I*Id1+Q*Qd1 : Subsystem
  IQ_Delay : Subsystem
  I^2+Q^2 : Subsystem
  Q*Id1-I*Qd1 : Subsystem
  Reinterpret : xbsIndex_r4/Reinterpret  force_arith_type=on  arith_type=Unsigned  force_bin_pt=on  bin_pt=0  block_type=reinterpret
      settings: infoedit="Changes signal type without altering the binary representation.   You can changed the signal between signed and unsigned, and relocate the binary point.<P><P>Hardware notes: In hardware this block costs nothing.<P><P>Example:  Suppose the input is 6 bits wide, signed, with 2 fractional bits, and the output is forced to unsigned with 0 fractional bits.  Then an input of -2.0 (1110.00 in binary 2's complement) becomes an output of 56 (111000 in binary)."  block_version=8.2
  Reinterpret1 : xbsIndex_r4/Reinterpret  force_arith_type=on  arith_type=Unsigned  force_bin_pt=on  bin_pt=0  block_type=reinterpret
      settings: infoedit="Changes signal type without altering the binary representation.   You can changed the signal between signed and unsigned, and relocate the binary point.<P><P>Hardware notes: In hardware this block costs nothing.<P><P>Example:  Suppose the input is 6 bits wide, signed, with 2 fractional bits, and the output is forced to unsigned with 0 fractional bits.  Then an input of -2.0 (1110.00 in binary 2's complement) becomes an output of 56 (111000 in binary)."  block_version=8.2
  IQ_Data : Outport
  A Data : Outport  Port=2
  B_Data : Outport  Port=3
  P_Data : Outport  Port=4
  M_Out : Outport  Port=5
  N_Out : Outport  Port=6
  Gate1_Out : Outport  Port=7
  Gate2_Out : Outport  Port=8
  Reset_Out : Outport  Port=9
  IQ Index_Out : Outport  Port=10
  IQ Length_Out : Outport  Port=11
  wires:
  Gate1_In/1 -> Delay/1, IQ_Delay/2(Gate1)
  Gate2_In/1 -> Delay3/1, IQ_Delay/3(Gate2)
  I^2+Q^2/1(P) -> P_Data/1
  I*Id1+Q*Qd1/1(A) -> A Data/1
  Q*Id1-I*Qd1/1(B) -> B_Data/1
  Delay/1 -> Gate1_Out/1
  Delay3/1 -> Gate2_Out/1
  M/1 -> M_Out/1
  N/1 -> N_Out/1
  Concat/1 -> Delay4/1, IQ_Delay/1(IQ_In)
  Reinterpret/1 -> Concat/1
  Reinterpret1/1 -> Concat/2
  Reset_In/1 -> Reset_Out/1, IQ_Delay/4(Reset)
  Delay1/1 -> I*Id1+Q*Qd1/1(I), Q*Id1-I*Qd1/3(I), I^2+Q^2/1(I)
  Delay2/1 -> I*Id1+Q*Qd1/3(Q), Q*Id1-I*Qd1/1(Q), I^2+Q^2/2(Q)
  IQ_Delay/1(I Delay Out) -> I*Id1+Q*Qd1/2(I Delay 1), Q*Id1-I*Qd1/2(I Delay 1)
  IQ_Delay/2(Q Delay Out) -> I*Id1+Q*Qd1/4(Q Delay 1), Q*Id1-I*Qd1/4(Q Delay 1)
  Delay4/1 -> IQ_Data/1
  IQ Index/1 -> IQ Index_Out/1
  IQ Length/1 -> IQ Length_Out/1
  I/1 -> Reinterpret/1, Delay1/1
  Q/1 -> Delay2/1, Reinterpret1/1

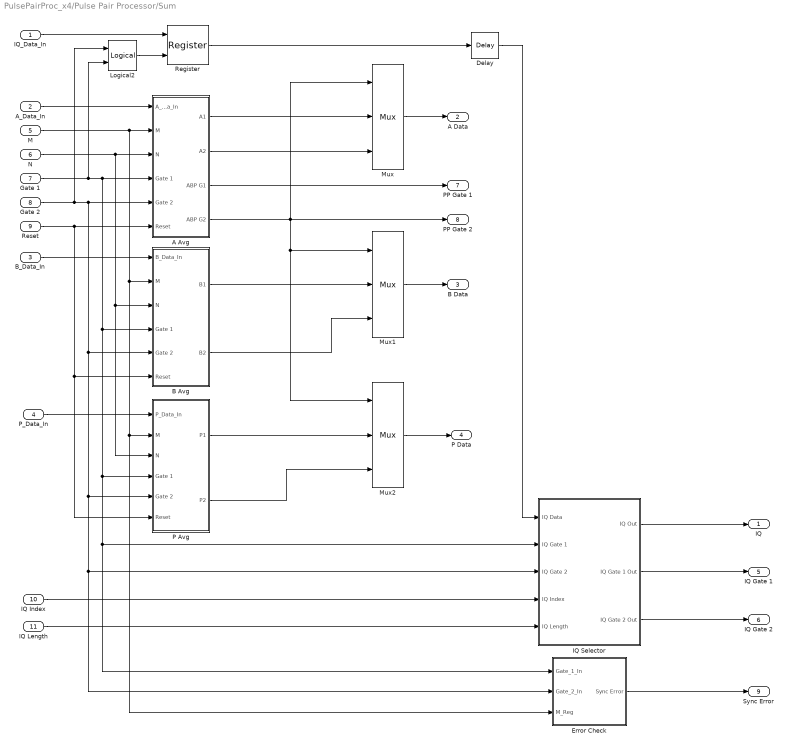
== system PulsePairProc_x4/Pulse Pair Processor/Sum ==
  IQ_Data_In : Inport
  A_Data_In : Inport  Port=2
  B_Data_In : Inport  Port=3
  P_Data_In : Inport  Port=4
  M : Inport  Port=5
  N : Inport  Port=6
  Gate 1 : Inport  Port=7
  Gate 2 : Inport  Port=8
  Reset : Inport  Port=9
  IQ Index : Inport  Port=10
  IQ Length : Inport  Port=11
  A Avg : Subsystem
  B Avg : Subsystem
  Delay : xbsIndex_r4/Delay  en=off  latency=2  dbl_ovrd=off  reg_retiming=off  block_type=delay
      settings: infoedit=Hardware notes: A delay line is a chain, each link of which is an SRL16 followed by a flip-flop. If register retiming is enabled, the delay line is a chain of flip-flops.  block_version=8.2
  Error Check : Subsystem
  IQ Selector : Subsystem
  Logical2 : xbsIndex_r4/Logical  logical_function=NOR  inputs=2  en=off  latency=0  precision=Full  arith_type=Unsigned  n_bits=16  bin_pt=0  align_bp=on  dbl_ovrd=off  block_type=logical
      settings: block_version=8.2
  Mux : xbsIndex_r4/Mux  inputs=2  en=off  latency=0  precision=Full  arith_type=Unsigned  n_bits=16  bin_pt=14  quantization=Truncate  overflow=Wrap  dbl_ovrd=off  block_type=mux
      settings: block_version=8.2
  Mux1 : xbsIndex_r4/Mux  inputs=2  en=off  latency=0  precision=Full  arith_type=Unsigned  n_bits=16  bin_pt=14  quantization=Truncate  overflow=Wrap  dbl_ovrd=off  block_type=mux
      settings: block_version=8.2
  Mux2 : xbsIndex_r4/Mux  inputs=2  en=off  latency=0  precision=Full  arith_type=Unsigned  n_bits=16  bin_pt=14  quantization=Truncate  overflow=Wrap  dbl_ovrd=off  block_type=mux
      settings: block_version=8.2
  P Avg : Subsystem
  Register : xbsIndex_r4/Register  init=0  rst=on  en=off  dbl_ovrd=off  block_type=register
      settings: block_version=8.2
  IQ : Outport
  A Data : Outport  Port=2
  B Data : Outport  Port=3
  P Data : Outport  Port=4
  IQ Gate 1 : Outport  Port=5
  IQ Gate 2 : Outport  Port=6
  PP Gate 1 : Outport  Port=7
  PP Gate 2 : Outport  Port=8
  Sync Error : Outport  Port=9
  wires:
  A_Data_In/1 -> A Avg/1(A_Data_In)
  M/1 -> A Avg/2(M), B Avg/2(M), P Avg/2(M), Error Check/3(M_Reg)
  N/1 -> A Avg/3(N), B Avg/3(N), P Avg/3(N)
  Gate 1/1 -> A Avg/4(Gate 1), B Avg/4(Gate 1), P Avg/4(Gate 1), IQ Selector/2(IQ Gate 1), Error Check/1(Gate_1_In), Logical2/2
  Gate 2/1 -> A Avg/5(Gate 2), B Avg/5(Gate 2), P Avg/5(Gate 2), IQ Selector/3(IQ Gate 2), Error Check/2(Gate_2_In), Logical2/1
  B_Data_In/1 -> B Avg/1(B_Data_In)
  P_Data_In/1 -> P Avg/1(P_Data_In)
  A Avg/3(ABP G1) -> PP Gate 1/1
  A Avg/4(ABP G2) -> PP Gate 2/1, Mux/1, Mux1/1, Mux2/1
  Reset/1 -> A Avg/6(Reset), B Avg/6(Reset), P Avg/6(Reset)
  IQ_Data_In/1 -> Register/1
  Logical2/1 -> Register/2
  Mux/1 -> A Data/1
  A Avg/1(A1) -> Mux/2
  A Avg/2(A2) -> Mux/3
  Mux1/1 -> B Data/1
  B Avg/1(B1) -> Mux1/2
  B Avg/2(B2) -> Mux1/3
  Mux2/1 -> P Data/1
  P Avg/1(P1) -> Mux2/2
  P Avg/2(P2) -> Mux2/3
  IQ Selector/1(IQ Out) -> IQ/1
  IQ Index/1 -> IQ Selector/4(IQ Index)
  IQ Length/1 -> IQ Selector/5(IQ Length)
  IQ Selector/2(IQ Gate 1 Out) -> IQ Gate 1/1
  IQ Selector/3(IQ Gate 2 Out) -> IQ Gate 2/1
  Register/1 -> Delay/1
  Delay/1 -> IQ Selector/1(IQ Data)
  Error Check/1(Sync Error) -> Sync Error/1
